simulink model "Controller"  (R2026a)
settings: Solver=VariableStepAuto
settings Model: Creator=pikha  LastModifiedBy=pikha

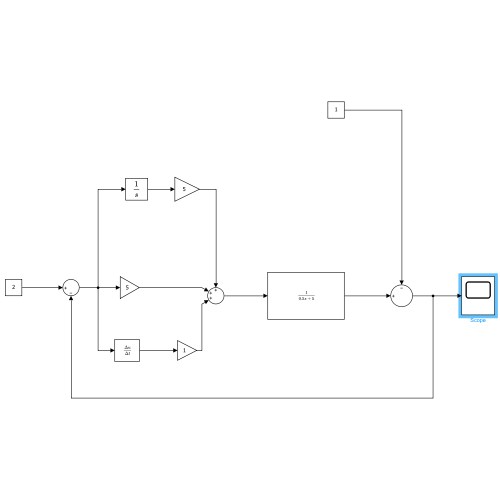
[thumbnail: Simulink's stored preview of the top-level diagram]
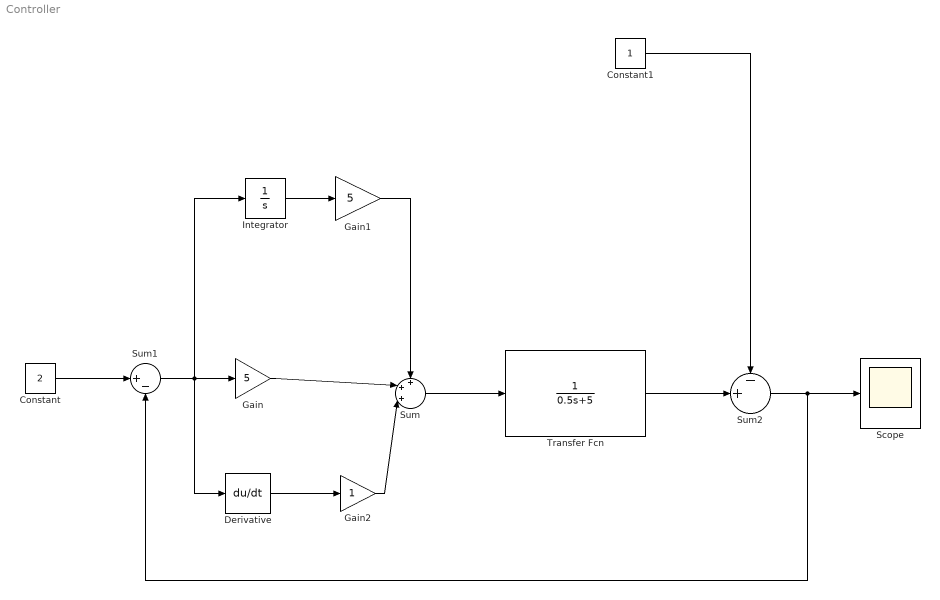
== system Controller ==
  Constant : Constant  Value=2
  Constant1 : Constant
  Derivative : Derivative
  Gain : Gain  Gain=5
  Gain1 : Gain  Gain=5
  Gain2 : Gain
  Integrator : Integrator
  Scope : Scope
      settings: ActiveDisplayYMinimum=-1.3743257184691515  ActiveDisplayYMaximum=2.3689314662223637
  Sum : Sum  Inputs=+++|
  Sum1 : Sum  Inputs=|+-
  Sum2 : Sum  Inputs=-+|
  Transfer Fcn : TransferFcn  Denominator=[0.5 5]
  wires:
  Sum1/1 -> Derivative/1, Integrator/1, Gain/1
  Integrator/1 -> Gain1/1
  Gain1/1 -> Sum/1
  Gain/1 -> Sum/2
  Gain2/1 -> Sum/3
  Sum/1 -> Transfer Fcn/1
  Constant/1 -> Sum1/1
  Derivative/1 -> Gain2/1
  Constant1/1 -> Sum2/1
  Transfer Fcn/1 -> Sum2/2
  Sum2/1 -> Scope/1, Sum1/2
